simulink library "CAN_out_lib"  (R2016b)
settings: Solver=VariableStepAuto  StartTime=0.0  StopTime=10.0  RelTol=1e-3
undefined symbols (not defined in the file): body_rates, fsw_params, gyro_valid, mag_eci_unit, pos_eci_km, quat_cmd, sc_above_gs, sc_in_sun, sc_mode, sc_quat, vel_eci_kmps, vel_point
libraries: bus_stubs_fsw x1, quat_degerr_check x1
settings Model: Creator=taylorreynolds  LastModifiedBy=Taylor

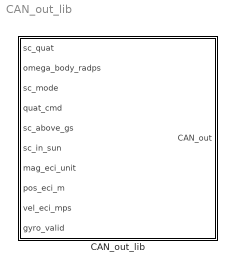
== system CAN_out_lib ==
  CAN_out_lib : Subsystem

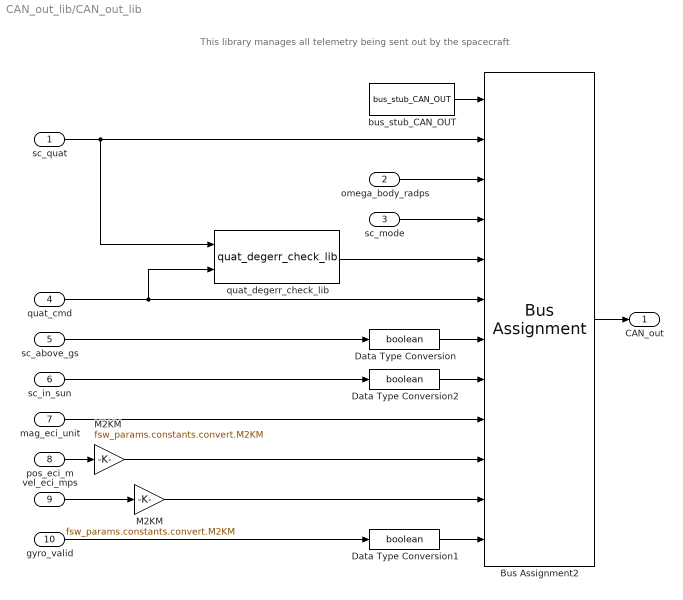
== system CAN_out_lib/CAN_out_lib ==
  note: This library manages all telemetry being sent out by the spacecraft
  sc_quat : Inport
  omega_body_radps : Inport  Port=2
  sc_mode : Inport  Port=3
  quat_cmd : Inport  Port=4
  sc_above_gs : Inport  Port=5
  sc_in_sun : Inport  Port=6
  mag_eci_unit : Inport  Port=7
  pos_eci_m : Inport  Port=8
  vel_eci_mps : Inport  Port=9
  gyro_valid : Inport  Port=10
  Bus Assignment2 : BusAssignment  AssignedSignals=sc_quat,body_rates,sc_mode,vel_point,quat_cmd,sc_above_gs,sc_in_sun,mag_eci_unit,pos_eci_km,vel_eci_kmps,gyro_valid
  Data Type Conversion : DataTypeConversion  OutDataTypeStr=boolean
  Data Type Conversion1 : DataTypeConversion  OutDataTypeStr=boolean
  Data Type Conversion2 : DataTypeConversion  OutDataTypeStr=boolean
  M2KM : Gain  Gain=fsw_params.constants.convert.M2KM
  "M2KM " : Gain  Gain=fsw_params.constants.convert.M2KM
  bus_stub_CAN_OUT : bus_stubs_fsw/bus_stub_CAN_OUT
  quat_degerr_check_lib : quat_degerr_check/quat_degerr_check_lib  point_tol=fsw_params.bus.point_tol
  CAN_out : Outport
  wires:
  bus_stub_CAN_OUT/1 -> Bus Assignment2/1
  Bus Assignment2/1 -> CAN_out/1
  sc_above_gs/1 -> Data Type Conversion/1
  sc_quat/1 -> quat_degerr_check_lib/1, Bus Assignment2/2
  omega_body_radps/1 -> Bus Assignment2/3
  sc_mode/1 -> Bus Assignment2/4
  quat_cmd/1 -> quat_degerr_check_lib/2, Bus Assignment2/6
  quat_degerr_check_lib/1 -> Bus Assignment2/5
  Data Type Conversion1/1 -> Bus Assignment2/12
  gyro_valid/1 -> Data Type Conversion1/1
  sc_in_sun/1 -> Data Type Conversion2/1
  pos_eci_m/1 -> "M2KM "/1
  vel_eci_mps/1 -> M2KM/1
  M2KM/1 -> Bus Assignment2/11
  "M2KM "/1 -> Bus Assignment2/10
  mag_eci_unit/1 -> Bus Assignment2/9
  Data Type Conversion2/1 -> Bus Assignment2/8
  Data Type Conversion/1 -> Bus Assignment2/7
